simulink model "AW_test"  (R2015a)
settings: Solver=ode5  StartTime=0.0  StopTime=80  FixedStep=5e-5  MaxStep=5e-5  RelTol=1e-3
values from neighbouring files (symbols this model uses):
  F = [-58.0981835397 -4179.57477778 -14.3009592549 -19.6551859971 -26.1377959927 51.7079073443 78.2309892718 -133.106022928 -125.54564289 -182.0885271 37.0670033238 40.9567129567 ... (144 elements, 12x12)]    [controller.mat]    (also in main_matlab_Corollary1.m = rlqg.A; main_matlab_Theorem3.m = rlqg.A; main_matlab_Theorem4.m = rlqg.A)
  G = [0.70645219319 -0.459324928491 1.97272580341 3.24573294172 13.9295718254 5.65537256369 -43.2723544643 48.5060616978 79.1032122304 114.834038365 0.0916332028948 -11.1940741965]    [controller.mat]    (also in main_matlab_Corollary1.m = rlqg.B; main_matlab_Theorem3.m = rlqg.B; main_matlab_Theorem4.m = rlqg.B)
  H = [64.5329237696 -12.8289022427 -137.386503701 73.2919038483 43.4280804178 151.107833676 54.9118478641 123.622857411 -29.577337272 16.1677085133 -56.2730534034 204.335066283 ... (24 elements, 2x12)]    [controller.mat]    (also in identified_t1.mat = [-0.00603819148621 -0.0121645329261 0.00178372873077 -0.0204; main_matlab_Corollary1.m = rlqg.C; main_matlab_Theorem3.m = rlqg.C; main_matlab_Theorem4.m = rlqg.C)
  L = [0 0]    [controller.mat]    (also in main_matlab_Corollary1.m = rlqg.D; main_matlab_Theorem3.m = rlqg.D; main_matlab_Theorem4.m = rlqg.D)
  M = inv(Q1)*Y    [main_matlab_Corollary1.m]    (also in main_matlab_Theorem3.m; main_matlab_Theorem4.m)
undefined symbols (not defined in the file or in its folder): Af, Bf, Cf, Hf
libraries: simulink x1
settings Model: Creator=p4wp4w  LastModifiedBy=Ablah

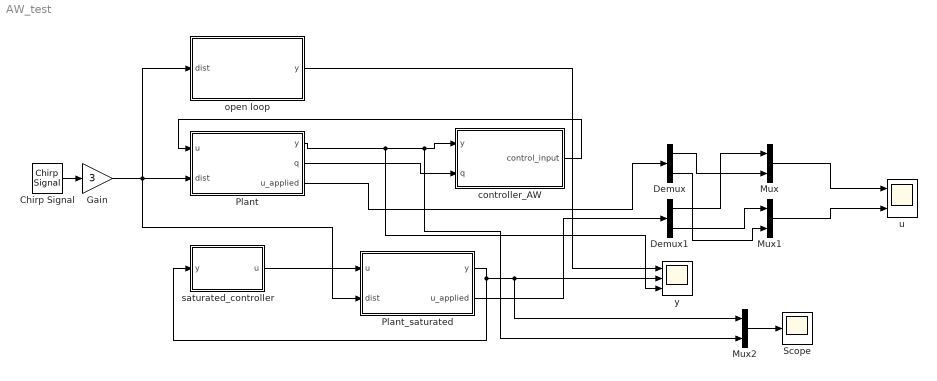
== system AW_test ==
  Chirp Signal : simulink/Sources/Chirp Signal  f1=0.1  T=80  f2=800
  Demux : Demux  Outputs=2
  Demux1 : Demux  Outputs=2
  Gain : Gain  Gain=3
  Mux : Mux  Inputs=2
  Mux1 : Mux  Inputs=2
  Mux2 : Mux  Inputs=2
  Plant : Subsystem
  Plant_saturated : Subsystem
  Scope : Scope
      settings: SaveName=ScopeData4
  controller_AW : Subsystem
  open loop : Subsystem
  "saturated_controller " : Subsystem
  u : Scope  NumInputPorts=2
      settings: ShowLegends=on  YMin=-0.45~-0.2  YMax=0.2~0.125
  y : Scope  NumInputPorts=3
      settings: YMin=-0.03~-0.03~-0.035  YMax=0.03~0.03~0.03
  wires:
  Plant/1(y) -> y/3, Mux2/2, controller_AW/1(y)
  Plant/2(q) -> controller_AW/2(q)
  controller_AW/1("control_input ") -> Plant/1(u)
  Chirp Signal/1 -> Gain/1
  "saturated_controller "/1(u) -> Plant_saturated/1(u)
  Plant_saturated/1(y) -> Mux2/1, y/2, "saturated_controller "/1(y)
  Demux1/1 -> Mux/1
  Demux/1 -> Mux/2
  Demux1/2 -> Mux1/1
  Demux/2 -> Mux1/2
  Mux/1 -> u/1
  Mux1/1 -> u/2
  Plant_saturated/2(u_applied) -> Demux1/1
  Plant/3(u_applied) -> Demux/1
  Gain/1 -> Plant_saturated/2(dist), open loop/1(dist), Plant/2(dist)
  open loop/1(y) -> y/1
  Mux2/1 -> Scope/1

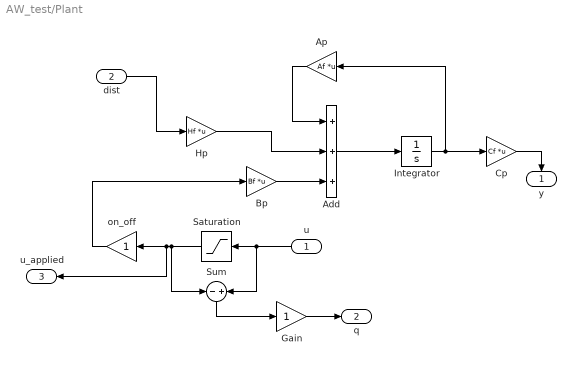
== system AW_test/Plant ==
  u : Inport
  dist : Inport  Port=2
  Add : Sum  Inputs=+++
  Ap : Gain  Gain=Af  Multiplication=Matrix(K*u)
  Bp : Gain  Gain=Bf  Multiplication=Matrix(K*u)
  Cp : Gain  Gain=Cf  Multiplication=Matrix(K*u)
  Gain : Gain
  Hp : Gain  Gain=Hf  Multiplication=Matrix(K*u)
  Integrator : Integrator
  Saturation : Saturate  UpperLimit=100  LowerLimit=-100
  Sum : Sum  Inputs=-|+
  on_off : Gain
  y : Outport
  q : Outport  Port=2
  u_applied : Outport  Port=3
  wires:
  Add/1 -> Integrator/1
  Cp/1 -> y/1
  Hp/1 -> Add/2
  on_off/1 -> Bp/1
  Integrator/1 -> Cp/1, Ap/1
  Saturation/1 -> Sum/1, on_off/1, u_applied/1
  Ap/1 -> Add/1
  u/1 -> Sum/2, Saturation/1
  Bp/1 -> Add/3
  Sum/1 -> Gain/1
  dist/1 -> Hp/1
  Gain/1 -> q/1

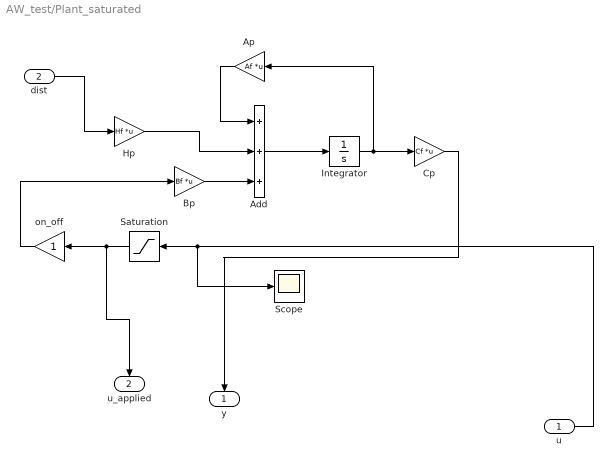
== system AW_test/Plant_saturated ==
  u : Inport
  dist : Inport  Port=2
  Add : Sum  Inputs=+++
  Ap : Gain  Gain=Af  Multiplication=Matrix(K*u)
  Bp : Gain  Gain=Bf  Multiplication=Matrix(K*u)
  Cp : Gain  Gain=Cf  Multiplication=Matrix(K*u)
  Hp : Gain  Gain=Hf  Multiplication=Matrix(K*u)
  Integrator : Integrator
  Saturation : Saturate  UpperLimit=100  LowerLimit=-100
  Scope : Scope
      settings: YMin=-10  YMax=10  SaveName=ScopeData2
  on_off : Gain
  y : Outport
  u_applied : Outport  Port=2
  wires:
  dist/1 -> Hp/1
  Bp/1 -> Add/3
  u/1 -> Scope/1, Saturation/1
  Ap/1 -> Add/1
  Saturation/1 -> u_applied/1, on_off/1
  Integrator/1 -> Ap/1, Cp/1
  on_off/1 -> Bp/1
  Hp/1 -> Add/2
  Cp/1 -> y/1
  Add/1 -> Integrator/1

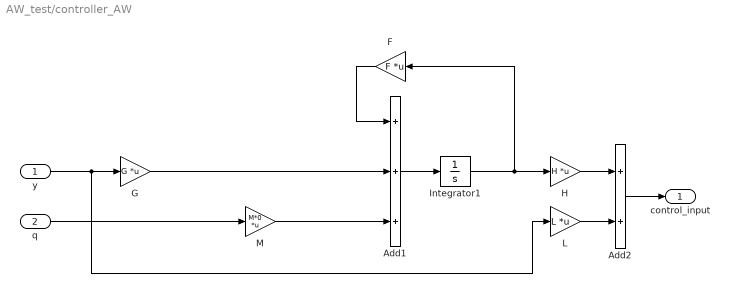
== system AW_test/controller_AW ==
  y : Inport
  q : Inport  Port=2
  Add1 : Sum  Inputs=+++
  Add2 : Sum
  F : Gain  Gain=F  Multiplication=Matrix(K*u)
  G : Gain  Gain=G  Multiplication=Matrix(K*u)
  H : Gain  Gain=H  Multiplication=Matrix(K*u)
  Integrator1 : Integrator
  L : Gain  Gain=L  Multiplication=Matrix(K*u)
  M : Gain  Gain=M*0  Multiplication=Matrix(K*u)
  "control_input " : Outport
  wires:
  H/1 -> Add2/1
  Add1/1 -> Integrator1/1
  F/1 -> Add1/1
  G/1 -> Add1/2
  Integrator1/1 -> H/1, F/1
  L/1 -> Add2/2
  Add2/1 -> "control_input "/1
  y/1 -> L/1, G/1
  q/1 -> M/1
  M/1 -> Add1/3

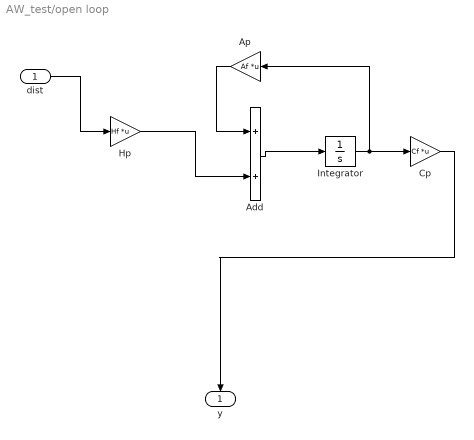
== system AW_test/open loop ==
  dist : Inport
  Add : Sum
  Ap : Gain  Gain=Af  Multiplication=Matrix(K*u)
  Cp : Gain  Gain=Cf  Multiplication=Matrix(K*u)
  Hp : Gain  Gain=Hf  Multiplication=Matrix(K*u)
  Integrator : Integrator
  y : Outport
  wires:
  dist/1 -> Hp/1
  Ap/1 -> Add/1
  Integrator/1 -> Ap/1, Cp/1
  Hp/1 -> Add/2
  Cp/1 -> y/1
  Add/1 -> Integrator/1

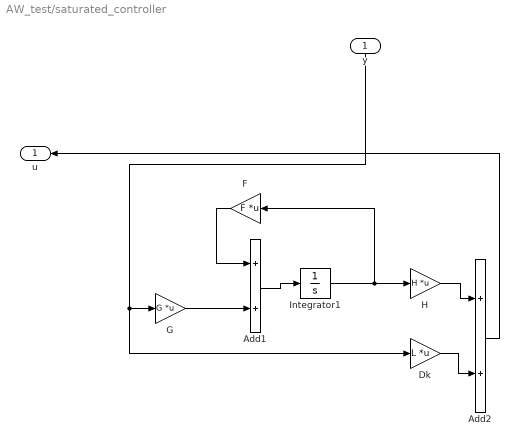
== system AW_test/saturated_controller  ==
  y : Inport
  Add1 : Sum
  Add2 : Sum
  Dk : Gain  Gain=L  Multiplication=Matrix(K*u)
  F : Gain  Gain=F  Multiplication=Matrix(K*u)
  G : Gain  Gain=G  Multiplication=Matrix(K*u)
  "H " : Gain  Gain=H  Multiplication=Matrix(K*u)
  Integrator1 : Integrator
  u : Outport
  wires:
  G/1 -> Add1/2
  Add1/1 -> Integrator1/1
  "H "/1 -> Add2/1
  Dk/1 -> Add2/2
  Integrator1/1 -> "H "/1, F/1
  Add2/1 -> u/1
  F/1 -> Add1/1
  y/1 -> Dk/1, G/1
